simulink model "on_line_ciagly_zmienny_18"  (R2018b)
settings: Solver=FixedStepAuto  StartTime=0.0  StopTime=20  FixedStep=0.1  RelTol=1e-3
model workspace (MAT data in the model file):
  denom = Simulink.Parameter
  denom.Value = [1 0.3 0.4]
  denom.DataType = 'auto'
  denom.Dimensions = [1 3]
libraries: ctrlSharedLib x1, cstblocks x1
settings Model: Creator=Dominik  LastModifiedBy=user
settings SFSimCC: SimUseLocalCustomCode=off
settings RTWCC: RTWUseLocalCustomCode=off

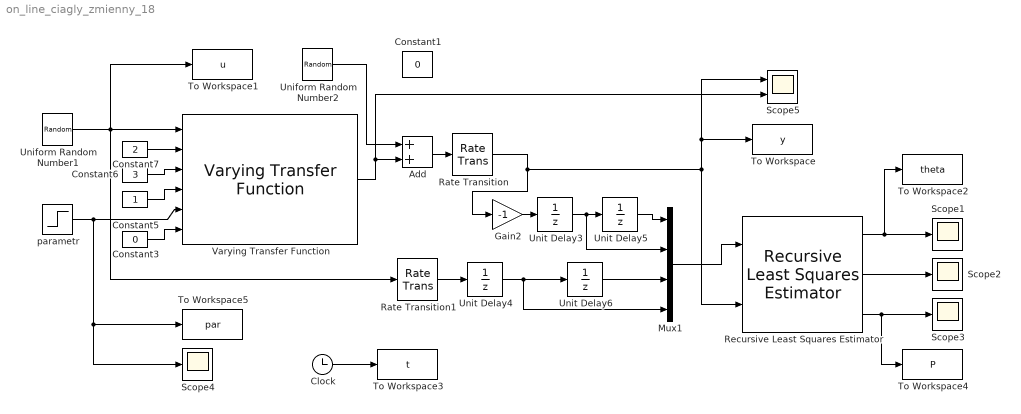
== system on_line_ciagly_zmienny_18 ==
  Add : Sum
  Clock : Clock
  Constant1 : Constant  Value=0
  Constant3 : Constant  Value=0
  Constant5 : Constant
  Constant6 : Constant  Value=3
  Constant7 : Constant  Value=2
  Gain2 : Gain  Gain=-1
  Mux1 : Mux
  Rate Transition : RateTransition  OutPortSampleTime=0.1
  Rate Transition1 : RateTransition
  Recursive Least Squares Estimator : ctrlSharedLib/Recursive Least Squares Estimator  InitialEstimateSource=None  InitialParameterData=4  P0=10000  InitialRegressors=0  InitialOutputs=0  History=Infinite  WindowLength=200  EstimationMethod=Forgetting Factor  AdaptationParameter=0.98  HasTimeVaryingAdaptationParameter=off  NormalizationBias=eps  OutputError=on  OutputP=on  AddEnablePort=off  InputProcessing=Sample-based  Ts=-1
      settings: SourceProductName=Control System Toolbox  SourceProductBaseCode=CT
  Scope{1..4} (4 alike) : Scope
  Scope5 : Scope  NumInputPorts=2
  To Workspace : ToWorkspace  VariableName=y  SampleTime=-1
  To Workspace1 : ToWorkspace  VariableName=u  SampleTime=-1
  To Workspace2 : ToWorkspace  VariableName=theta  SampleTime=-1
  To Workspace3 : ToWorkspace  VariableName=t  SampleTime=-1
  To Workspace4 : ToWorkspace  VariableName=P  SampleTime=-1
  To Workspace5 : ToWorkspace  VariableName=par  SampleTime=-1
  Uniform Random Number1 : UniformRandomNumber  SampleTime=0.1
  Uniform Random Number2 : UniformRandomNumber  Minimum=-0.005  Maximum=0.005  Seed=3124212  SampleTime=0.1
  Unit Delay{3..6} (4 alike) : UnitDelay  SampleTime=-1
  Varying Transfer Function : cstblocks/Linear Parameter Varying/Varying Transfer Function  N=2
      settings: SourceProductName=Control System Toolbox
  parametr : Step  Time=10  Before=2  After=1.5  SampleTime=0
  wires:
  Recursive Least Squares Estimator/1 -> Scope1/1, To Workspace2/1
  Clock/1 -> To Workspace3/1
  Recursive Least Squares Estimator/2 -> Scope2/1
  Recursive Least Squares Estimator/3 -> To Workspace4/1, Scope3/1
  Unit Delay3/1 -> Mux1/2, Unit Delay5/1
  Gain2/1 -> Unit Delay3/1
  Unit Delay5/1 -> Mux1/1
  Mux1/1 -> Recursive Least Squares Estimator/1
  Unit Delay4/1 -> Mux1/4, Unit Delay6/1
  Unit Delay6/1 -> Mux1/3
  Uniform Random Number1/1 -> Rate Transition1/1, Varying Transfer Function/1, To Workspace1/1
  Uniform Random Number2/1 -> Add/1
  Varying Transfer Function/1 -> Add/2, Scope5/2
  Rate Transition/1 -> Scope5/1, To Workspace/1, Recursive Least Squares Estimator/2, Gain2/1
  Rate Transition1/1 -> Unit Delay4/1
  Add/1 -> Rate Transition/1
  Constant3/1 -> Varying Transfer Function/6
  parametr/1 -> Varying Transfer Function/5, Scope4/1, To Workspace5/1
  Constant5/1 -> Varying Transfer Function/4
  Constant7/1 -> Varying Transfer Function/2
  Constant6/1 -> Varying Transfer Function/3
